simulink model "sampleModel1471_5_sub_sub"  (R2023a)
settings: Solver=VariableStepAuto  StartTime=0.0  StopTime=10.0  RelTol=1e-3
libraries: simulink x5, hdlsllib x2
settings Model: Creator=user1  LastModifiedBy=user1
settings OptimizationCC: BlockReduction=off  ConditionallyExecuteInputs=off

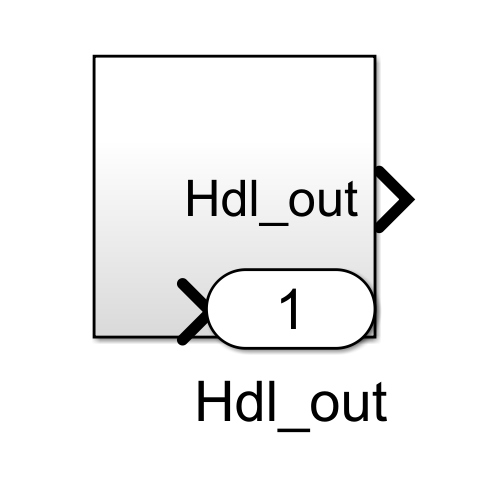
[thumbnail: Simulink's stored preview of the top-level diagram]
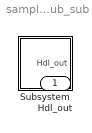
== system sampleModel1471_5_sub_sub ==
  Subsystem : Subsystem
  Hdl_out : Outport  OutDataTypeStr=uint8

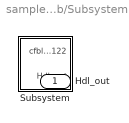
== system sampleModel1471_5_sub_sub/Subsystem ==
  Subsystem : Subsystem
  Hdl_out : Outport  OutDataTypeStr=uint8

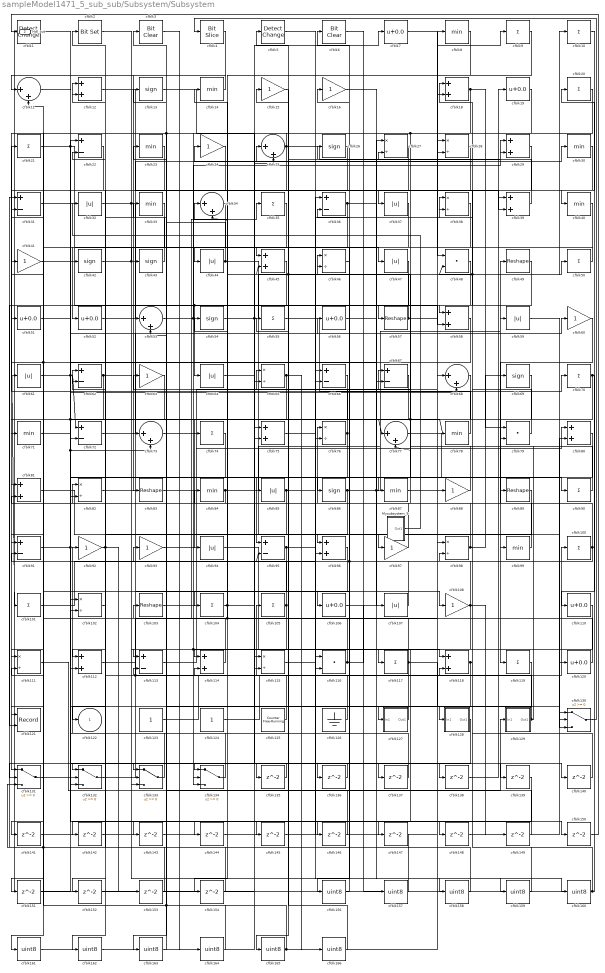
== system sampleModel1471_5_sub_sub/Subsystem/Subsystem ==
  Mysubsystem_9 : Subsystem  TreatAsAtomicUnit=on  RTWFcnName=Mysubsystem_9
      settings: RTWFcnNameOpts=User specified  RTWFileNameOpts=Use function name
  cfblk1 : simulink/Logic and Bit Operations/Detect Change  vinit=0  OutDataTypeStr=uint8
      settings: LibrarySourceBlock=|
      | hdlsllib/Logic and Bit
      | Operations/Detect
      | Change
  cfblk{9..10,20..21,35,50,55,70,74,90,100..101,104..105,117,119} (16 alike) : Sum  Inputs=+  OutDataTypeStr=uint8
  cfblk{27..28,38,46,65,76,82,98,102,111,115} (11 alike) : Product  Inputs=*/  OutDataTypeStr=uint8  RndMeth=Zero  SaturateOnIntegerOverflow=on
  cfblk{49,57,83,89,103} (5 alike) : Reshape
  cfblk{7,19,51..52,56,106,110,120} (8 alike) : Bias  Bias=0.0  SaturateOnIntegerOverflow=off
  cfblk{32,37,44,47,59,61,64,85,94,107} (10 alike) : Abs  OutDataTypeStr=uint8  SaturateOnIntegerOverflow=off
  cfblk{15..16,24,41,60,63,88,92..93,97,108} (11 alike) : Gain  OutDataTypeStr=uint8
  cfblk{11,25,34,53,68,73,77} (7 alike) : Sum  Inputs=|++  OutDataTypeStr=uint8
  cfblk{12,18,29,39,45,58,75,80..81,96,112,114,118} (13 alike) : Sum  OutDataTypeStr=uint8
  cfblk{22,31,36,62,66..67,72,91,95,113} (10 alike) : Sum  Inputs=+-  OutDataTypeStr=uint8
  cfblk116 : DotProduct  OutDataTypeStr=uint8
  cfblk121 : Record  FileSettingsInternal="{\"entries\":[{\"content\":{\"excelSettings\":{\"content\":{},\"type\":\"Streamout.ExcelSettings\"}},\"type\":\"Streamout.FileSettingStorage\",\"uuid\":\"\"}],\"packageUris\":[\"http:\\/\\/schema.mathworks.com\\/mf0\\/streamout_blocks\\/R2020a\"],\"version\":\"1.0\"}"  Layout=[1 1]  SignalsInternal="{\"entries\":[{\"content\":{\"signals\":[{\"content\":{\"blockPath\":[],\"dimensions\":[1],\"domain\":\"\",\"lineColor\":\"#a2142f\",\"plots\":[1],\"port\":1,\"signalID\":20024,\"signalName\":\"cfblk37\"},\"type\":\"RecordBlkView.Signal\",\"uuid\":\"\"},{\"content\":{\"blockPath\":[],\"dimensions\":[1],\"domain\":\"\",\"lineColor\":\"#139fff\",\"plots\":[1],\"port\":2,\"signalID\":20027,\"signalName\":\"cfblk45\"},\"type\":\"RecordBlkView.Signal\",\"uuid\":\"\"}]},\"type\":\"RecordBlkView.InputSignals\",\"uuid\":\"\"}],\"packageUris\":[\"http:\\/\\/schema.mathworks.com\\/mf0\\/streamout_blocks\\/R2020a\"],\"version\":\"1.0\"}"  VisualizationBindings="{\"xyplotplugin\":{\"info\":[{\"series\":[{\"bindingParametersList\":[{\"parameter\":\"X-Axis\",\"signalID\":20024,\"signalName\":\"cfblk37\"},{\"parameter\":\"Y-Axis\",\"signalID\":20027,\"signalName\":\"cfblk45\"}],\"seriesID\":60236}],\"subplotID\":1}]}}"  CompatibilityTag=XY  st=-1
  cfblk123 : Constant  OutDataTypeStr=uint8  SampleTime=-1
  cfblk124 : Constant  OutDataTypeStr=uint8  SampleTime=-1
  cfblk125 : hdlsllib/Sources/Counter Free-Running  NumBits=16  tsamp=-1
  cfblk126 : Ground
  cfblk127 : Subsystem
      settings: LibrarySourceBlock=|
      | hdlsllib/Ports &
      | Subsystems/Subsystem
  cfblk128 : Subsystem
      settings: LibrarySourceBlock=|
      | hdlsllib/Ports &
      | Subsystems/Subsystem
  cfblk129 : Subsystem
      settings: LibrarySourceBlock=|
      | hdlsllib/Ports &
      | Subsystems/Subsystem
  cfblk{13,26,42..43,54,69,86} (7 alike) : Signum
  cfblk{130..134} (5 alike) : Switch  OutDataTypeStr=uint8  SaturateOnIntegerOverflow=off  InputSameDT=off
  cfblk{135..154} (20 alike) : Delay  SampleTime=1
  cfblk{8,14,23,30,33,40,71,78,84,87,99} (11 alike) : MinMax  OutDataTypeStr=uint8
  cfblk{156..166} (11 alike) : DataTypeConversion  OutDataTypeStr=uint8  SaturateOnIntegerOverflow=off  RndMeth=Floor
  cfblk2 : simulink/Logic and Bit Operations/Bit Set  iBit=0
      settings: LibrarySourceBlock=|
      | hdlsllib/Logic and Bit
      | Operations/Bit Set
  cfblk3 : simulink/Logic and Bit Operations/Bit Clear  iBit=0
      settings: LibrarySourceBlock=|
      | hdlsllib/Logic and Bit
      | Operations/Bit Clear
  cfblk4 : hdlsllib/Logic and Bit Operations/Bit Slice  lidx=7  ridx=0
  cfblk48 : DotProduct  OutDataTypeStr=uint8
  cfblk5 : simulink/Logic and Bit Operations/Detect Change  vinit=0  OutDataTypeStr=uint8
      settings: LibrarySourceBlock=|
      | hdlsllib/Logic and Bit
      | Operations/Detect
      | Change
  cfblk6 : simulink/Logic and Bit Operations/Bit Clear  iBit=0
      settings: LibrarySourceBlock=|
      | hdlsllib/Logic and Bit
      | Operations/Bit Clear
  cfblk79 : DotProduct  OutDataTypeStr=uint8
  cfblk122 : Outport  OutDataTypeStr=uint8  VectorParamsAs1DForOutWhenUnconnected=off
  Hdl_out : Outport  Port=2  OutDataTypeStr=uint8
  wires:
  Mysubsystem_9/1(Out1) -> cfblk32/1
  cfblk166/1 -> cfblk15/1
  cfblk165/1 -> cfblk13/1, cfblk98/1
  cfblk164/1 -> cfblk31/2, cfblk103/1
  cfblk163/1 -> cfblk3/1
  cfblk119/1 -> cfblk163/1
  cfblk162/1 -> cfblk115/2
  cfblk139/1 -> cfblk162/1
  cfblk161/1 -> cfblk115/1
  cfblk160/1 -> cfblk38/2, cfblk48/2, cfblk20/1, Hdl_out/1
  cfblk159/1 -> cfblk98/2
  cfblk2/1 -> cfblk159/1
  cfblk158/1 -> cfblk2/1
  cfblk56/1 -> cfblk158/1
  cfblk157/1 -> cfblk31/1, cfblk41/1
  cfblk156/1 -> cfblk6/1
  cfblk89/1 -> cfblk156/1
  cfblk154/1 -> cfblk22/1
  cfblk9/1 -> cfblk154/1
  cfblk153/1 -> cfblk111/2
  cfblk152/1 -> cfblk25/2
  cfblk151/1 -> cfblk82/2
  cfblk150/1 -> cfblk1/1
  cfblk149/1 -> cfblk113/2
  cfblk148/1 -> cfblk80/2
  cfblk147/1 -> cfblk131/3
  cfblk146/1 -> cfblk66/1
  cfblk145/1 -> cfblk96/2
  cfblk26/1 -> cfblk145/1
  cfblk144/1 -> cfblk65/2
  cfblk38/1 -> cfblk144/1
  cfblk143/1 -> cfblk116/1
  cfblk19/1 -> cfblk143/1
  cfblk142/1 -> cfblk28/1
  cfblk34/1 -> cfblk142/1
  cfblk141/1 -> cfblk68/1
  cfblk49/1 -> cfblk141/1
  cfblk140/1 -> cfblk118/2
  cfblk138/1 -> cfblk39/1
  cfblk64/1 -> cfblk138/1
  cfblk137/1 -> cfblk102/1
  cfblk11/1 -> cfblk137/1
  cfblk136/1 -> cfblk134/2
  cfblk135/1 -> cfblk131/2
  cfblk128/1(Out1) -> cfblk135/1
  cfblk54/1 -> cfblk10/1, cfblk7/1
  cfblk63/1 -> cfblk112/2
  cfblk96/1 -> cfblk111/1
  cfblk116/1 -> cfblk11/2, cfblk107/1
  cfblk12/1 -> cfblk39/2
  cfblk100/1 -> cfblk67/1, cfblk91/2
  cfblk117/1 -> cfblk22/2, cfblk34/2, cfblk114/2, cfblk130/3
  cfblk41/1 -> cfblk130/2
  cfblk10/1 -> cfblk40/1
  cfblk80/1 -> cfblk102/2
  cfblk22/1 -> cfblk91/1
  cfblk69/1 -> cfblk77/2, cfblk152/1
  cfblk102/1 -> cfblk82/1
  cfblk62/1 -> cfblk72/2, cfblk150/1
  cfblk59/1 -> cfblk130/1
  cfblk75/1 -> cfblk66/2
  cfblk110/1 -> cfblk127/1(In1)
  cfblk39/1 -> cfblk5/1
  cfblk51/1 -> cfblk78/1, cfblk139/1
  cfblk85/1 -> cfblk113/1, cfblk97/1
  cfblk29/1 -> cfblk87/1, cfblk77/1
  cfblk92/1 -> cfblk62/2, cfblk153/1
  cfblk30/1 -> cfblk58/1
  cfblk108/1 -> cfblk36/2, cfblk133/1, cfblk149/1
  cfblk126/1 -> cfblk12/2
  cfblk20/1 -> cfblk73/1, cfblk51/1, cfblk37/1
  cfblk91/1 -> cfblk42/1, cfblk133/3
  cfblk1/1 -> cfblk68/2
  cfblk42/1 -> cfblk44/1, cfblk76/2
  cfblk18/1 -> cfblk134/3, cfblk79/1
  cfblk129/1(Out1) -> cfblk25/1, cfblk45/2, cfblk79/2
  cfblk48/1 -> cfblk53/2
  cfblk120/1 -> cfblk34/1
  cfblk46/1 -> cfblk16/1
  cfblk90/1 -> cfblk63/1
  cfblk134/1 -> cfblk93/1
  cfblk105/1 -> cfblk54/1, cfblk133/2
  cfblk6/1 -> cfblk157/1
  cfblk24/1 -> cfblk132/3
  cfblk83/1 -> cfblk86/1
  cfblk33/1 -> cfblk52/1
  cfblk68/1 -> cfblk85/1
  cfblk65/1 -> cfblk94/1, cfblk166/1
  cfblk7/1 -> cfblk48/1
  cfblk86/1 -> cfblk19/1, cfblk29/1, cfblk122/1
  cfblk98/1 -> cfblk33/1, cfblk69/1
  cfblk112/1 -> cfblk28/2
  cfblk93/1 -> cfblk116/2, cfblk136/1
  cfblk53/1 -> cfblk29/2, cfblk140/1
  cfblk14/1 -> cfblk11/1
  cfblk104/1 -> cfblk128/1(In1), cfblk84/1
  cfblk71/1 -> cfblk73/2, cfblk146/1
  cfblk57/1 -> cfblk14/1, cfblk9/1
  cfblk127/1(Out1) -> cfblk46/2
  cfblk5/1 -> cfblk118/1
  cfblk4/1 -> cfblk43/1
  cfblk67/1 -> cfblk114/1
  cfblk84/1 -> cfblk59/1, cfblk81/2
  cfblk37/1 -> cfblk121/1
  cfblk81/1 -> cfblk120/1
  cfblk13/1 -> cfblk75/2
  cfblk101/1 -> cfblk36/1
  cfblk21/1 -> cfblk53/1, cfblk67/2
  cfblk35/1 -> cfblk83/1
  cfblk82/1 -> cfblk108/1
  cfblk43/1 -> cfblk12/1
  cfblk73/1 -> cfblk50/1
  cfblk61/1 -> cfblk72/1, cfblk89/1
  cfblk74/1 -> cfblk132/2
  cfblk16/1 -> cfblk99/1
  cfblk8/1 -> cfblk134/1
  cfblk97/1 -> cfblk76/1
  cfblk131/1 -> cfblk60/1
  cfblk107/1 -> cfblk95/2, cfblk26/1
  cfblk115/1 -> cfblk160/1
  cfblk36/1 -> cfblk104/1, cfblk148/1
  cfblk79/1 -> cfblk24/1
  cfblk95/1 -> cfblk38/1, cfblk161/1
  cfblk77/1 -> cfblk90/1
  cfblk132/1 -> cfblk75/1, cfblk8/1
  cfblk130/1 -> cfblk4/1
  cfblk103/1 -> cfblk80/1
  cfblk40/1 -> cfblk106/1
  cfblk3/1 -> cfblk164/1
  cfblk88/1 -> cfblk46/1
  cfblk76/1 -> cfblk95/1, cfblk55/1
  cfblk66/1 -> cfblk71/1
  cfblk70/1 -> cfblk110/1, cfblk74/1
  cfblk23/1 -> cfblk132/1
  cfblk52/1 -> cfblk30/1
  cfblk111/1 -> cfblk129/1(In1)
  cfblk124/1 -> cfblk100/1
  cfblk125/1 -> cfblk62/1
  cfblk28/1 -> cfblk81/1
  cfblk99/1 -> cfblk49/1
  cfblk72/1 -> cfblk56/1
  cfblk58/1 -> cfblk101/1, cfblk151/1
  cfblk78/1 -> cfblk21/1
  cfblk50/1 -> cfblk45/1
  cfblk87/1 -> cfblk88/1
  cfblk25/1 -> cfblk131/1, cfblk27/2, cfblk61/1
  cfblk113/1 -> cfblk65/1
  cfblk27/1 -> cfblk112/1
  cfblk123/1 -> cfblk18/2
  cfblk106/1 -> cfblk27/1
  cfblk118/1 -> cfblk18/1, cfblk147/1
  cfblk31/1 -> cfblk47/1
  cfblk15/1 -> cfblk165/1
  cfblk32/1 -> cfblk105/1, cfblk58/2
  cfblk60/1 -> cfblk119/1
  cfblk94/1 -> cfblk117/1
  cfblk133/1 -> cfblk92/1
  cfblk44/1 -> cfblk96/1, cfblk23/1
  cfblk114/1 -> cfblk35/1
  cfblk47/1 -> cfblk57/1
  cfblk45/1 -> cfblk64/1, cfblk121/2
  cfblk55/1 -> cfblk70/1

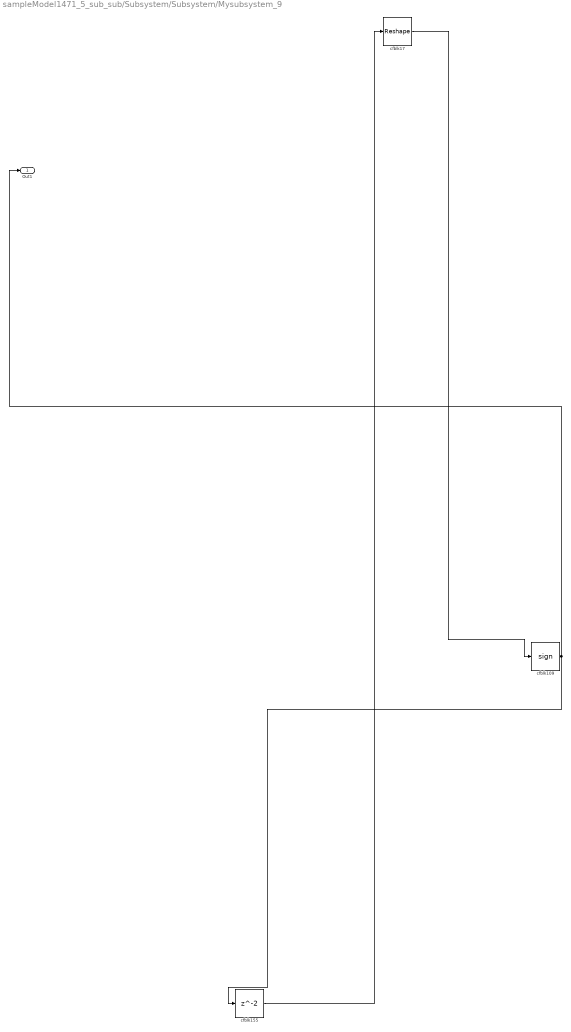
== system sampleModel1471_5_sub_sub/Subsystem/Subsystem/Mysubsystem_9 ==
  cfblk109 : Signum
  cfblk155 : Delay  SampleTime=1
  cfblk17 : Reshape
  Out1 : Outport
  wires:
  cfblk17/1 -> cfblk109/1
  cfblk109/1 -> Out1/1, cfblk155/1
  cfblk155/1 -> cfblk17/1

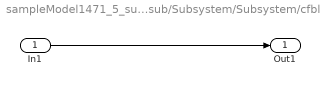
== system sampleModel1471_5_sub_sub/Subsystem/Subsystem/cfblk127 ==
  In1 : Inport
  Out1 : Outport
  wires:
  In1/1 -> Out1/1

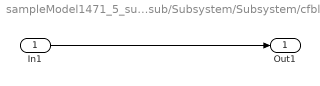
== system sampleModel1471_5_sub_sub/Subsystem/Subsystem/cfblk128 ==
  In1 : Inport
  Out1 : Outport
  wires:
  In1/1 -> Out1/1

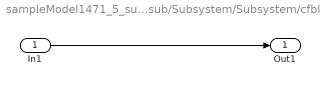
== system sampleModel1471_5_sub_sub/Subsystem/Subsystem/cfblk129 ==
  In1 : Inport
  Out1 : Outport
  wires:
  In1/1 -> Out1/1
